simulink model "temp"  (R2020a)
settings: Solver=VariableStepAuto  StartTime=0.0  StopTime=10.0  RelTol=1e-3
settings Model: Creator=faaizz  LastModifiedBy=faaizz

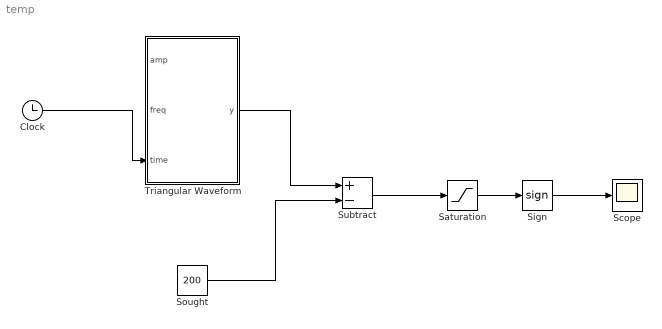
== system temp ==
  Clock : Clock
  Saturation : Saturate  UpperLimit=0  LowerLimit=-inf
  Scope : Scope
  Sign : Signum
  Sought : Constant  Value=200
  Subtract : Sum  Inputs=+-
  Triangular Waveform : MATLAB Function  TreatAsAtomicUnit=on
  wires:
  Clock/1 -> Triangular Waveform/3(time)
  Triangular Waveform/1(y) -> Subtract/1
  Sought/1 -> Subtract/2
  Subtract/1 -> Saturation/1
  Saturation/1 -> Sign/1
  Sign/1 -> Scope/1

== matlab function temp/Triangular Waveform ==
  data: amp input; freq input; y output; time input
function y = fcn(amp, freq, time)

% Period
T= 1/freq;
% Find posiiton in current period
t_pos= mod(time, T);
% Slope
m= amp/(T/2);

% Iutput sequence
y= zeros(size(time));

% Rising half
y(t_pos <= T/2)= m*t_pos(t_pos <= T/2);


% Falling half
y(t_pos > T/2)= amp - m*(t_pos(t_pos > T/2)-(T/2));

end
